simulink model "threelevel_12phase1"  (R2020b)
settings: Solver=FixedStepDiscrete  StartTime=0.0  StopTime=1  FixedStep=Ts_FEA  RelTol=1e-3
model workspace (MAT data in the model file):
  T_10kHz : Simulink.Parameter (value not decoded)
undefined symbols (not defined in the file): Cin, DiscIntNeverNeededParam, ESL, ESR, faif, Jm, kfeed_r, ki_n, kp_n, L, Ld, Line, Lq, ncmd_climb, ncmd_cruise, ncmd_run, ncmd_takeoff, p, Pcmd_climb, Pcmd_cruise, Pcmd_run, Pcmd_takeoff, Rs, Tcmd_run, Tcmd_start, Tcmd_time, time_climb, time_cruise, time_run, time_start, time_takeoff, Ts, Ts_Dead, Ts_FEA, Ts_speedloop, tswitch_climb, tswitch_takeoff, VDC, ws, zero_C1
libraries: powerlib x73, simulink x16, powerlib_meascontrol x16, slpidlib x13
(part 2 of 6)

== system threelevel_12phase1/CurrentLoop/Subsystem1/Subsystem ==
  ud : Inport
  uq : Inport  Port=2
  alpha : Inport  Port=3
  beta : Inport  Port=4
  dV : Inport  Port=5
  Atan2 : Trigonometry  Operator=atan2
  Constant : Constant
  Constant1 : Constant  Value=VDC
  Constant7 : Constant
  Divide : Product  Inputs=*/
  First_Order2 : Subsystem
  Gain : Gain  Gain=10
  PID Controller1 : slpidlib/PID Controller  Controller=PI  Form=Parallel  TimeDomain=Discrete-time  UseExternalTs=off  SampleTime=Ts  IntegratorMethod=Forward Euler  FilterMethod=Forward Euler  ControllerParametersSource=external  P=1/VDC  I=1/VDC  D=0  UseFilter=on  N=100  TunerSelectOption=Transfer Function Based (PID Tuner App)  InitialConditionSource=internal  InitialConditionForIntegrator=0  InitialConditionForFilter=0  DifferentiatorICPrevScaledInput=0  ExternalReset=none  TrackingMode=off  Kt=1  LimitOutput=on  SatLimitsSource=internal  UpperSaturationLimit=1  LowerSaturationLimit=-1  LinearizeAsGain=off  AntiWindupMode=none  Kb=1  POutMin=[]  POutMax=[]  IOutMin=[]  IOutMax=[]  DOutMin=[]  DOutMax=[]  NOutMin=[]  NOutMax=[]  SumOutMin=[]  SumOutMax=[]  SaturationOutMin=[]  SaturationOutMax=[]  PParamMin=[]  PParamMax=[]  IParamMin=[]  IParamMax=[]  DParamMin=[]  DParamMax=[]  NParamMin=[]  NParamMax=[]  KbParamMin=[]  KbParamMax=[]  KtParamMin=[]  KtParamMax=[]  KbOutMin=[]  KbOutMax=[]  KtOutMin=[]  KtOutMax=[]  IntegratorOutMin=[]  IntegratorOutMax=[]  FilterOutMin=[]  FilterOutMax=[]  SumI1OutMin=[]  SumI1OutMax=[]  SumI2OutMin=[]  SumI2OutMax=[]  SumI3OutMin=[]  SumI3OutMax=[]  SumI4OutMin=[]  SumI4OutMax=[]  SumDOutMin=[]  SumDOutMax=[]  DifferentiatorOutMin=[]  DifferentiatorOutMax=[]  FilterDiffOutCoefMin=[]  FilterDiffOutCoefMax=[]  ReciprocalOutMin=[]  ReciprocalOutMax=[]  SumDenOutMin=[]  SumDenOutMax=[]  SumNumOutMin=[]  SumNumOutMax=[]  DivideOutMin=[]  DivideOutMax=[]  UdiffTsProdOutMin=[]  UdiffTsProdOutMax=[]  NTsProdOutMin=[]  NTsProdOutMax=[]  UintegralTsProdOutMin=[]  UintegralTsProdOutMax=[]  UngainTsProdOutMin=[]  UngainTsProdOutMax=[]  IntegratorContinuousStateAttributes=''  IntegratorStateMustResolveToSignalObject=off  IntegratorRTWStateStorageClass=Auto  FilterContinuousStateAttributes=''  FilterStateMustResolveToSignalObject=off  FilterRTWStateStorageClass=Auto  ParallelPVariant=ExternalParameters  IdealPVariant=Disabled  IVariant=ExternalParameters  DVariant=Disabled  IntegratorVariant=Discrete  SatVariant=Enabled  AWVariant=Passthrough  PCopyVariant=Disabled  TRVariant=Disabled  FdbkBlocksVariant=Forward  IdealPFdbkVariant=Disabled  SatFdbkVariant=Disabled  DerivativeFilterVariant=Disabled  NVariant=Disabled  NCopyVariant=Disabled_SignalSpec  FilterICVariant=Disabled  IntegratorICVariant=InternalICs  ExternalResetVariant=Disabled  TRSumVariant=Passthrough  SumFdbkVariant=Disabled  SumVariant=Sum_PI  TsampFilterVariant=InternalTs  TsampNgainVariant=Passthrough  TsampIntegralVariant=Passthrough  ExternalSaturationOutDataTypeStr=Inherit: Same as second input
  Product1 : Product
  Saturation1 : Saturate  UpperLimit=1  LowerLimit=-1
  propose method1 : MATLAB Function  TreatAsAtomicUnit=on
  针对负载波动的P增量 : Subsystem  Commented=on
  r : Outport
  wires:
  Divide/1 -> Product1/1, Gain/1
  Constant1/1 -> Divide/2
  Constant7/1 -> Divide/1
  alpha/1 -> propose method1/2(alpha)
  uq/1 -> Atan2/2
  beta/1 -> propose method1/3(beta)
  propose method1/1(r) -> Saturation1/1
  Atan2/1 -> First_Order2/1(In1)
  ud/1 -> Atan2/1
  dV/1 -> PID Controller1/1
  Constant/1 -> Product1/2
  Gain/1 -> PID Controller1/3
  Product1/1 -> PID Controller1/2
  First_Order2/1(ADC_temp) -> propose method1/4(phi)
  Saturation1/1 -> r/1
  PID Controller1/1 -> propose method1/1(PI)

== system threelevel_12phase1/CurrentLoop/Subsystem1/Subsystem2 ==
  Compare : Inport
  AND13 : Logic  AllPortsSameDT=off  OutDataTypeStr=boolean
  AND14 : Logic  AllPortsSameDT=off  OutDataTypeStr=boolean
  Delay13 : Delay  DelayLength=Ts_Dead/Ts_FEA
  Demux : Demux  Outputs=6
  Demux1 : Demux  Outputs=6
  Mux : Mux  Inputs=12
  NOT6 : Logic  Operator=NOT  AllPortsSameDT=off  OutDataTypeStr=boolean
  NOT7 : Logic  Operator=NOT  AllPortsSameDT=off  OutDataTypeStr=boolean
  Output : Outport
  wires:
  Mux/1 -> Output/1
  Compare/1 -> Delay13/1, NOT6/1, AND13/1
  Delay13/1 -> NOT7/1, AND13/2
  NOT7/1 -> AND14/1
  NOT6/1 -> AND14/2
  AND13/1 -> Demux/1
  AND14/1 -> Demux1/1
  Demux/1 -> Mux/1
  Demux/2 -> Mux/2
  Demux/3 -> Mux/5
  Demux/4 -> Mux/6
  Demux/5 -> Mux/9
  Demux/6 -> Mux/10
  Demux1/1 -> Mux/3
  Demux1/2 -> Mux/4
  Demux1/3 -> Mux/7
  Demux1/4 -> Mux/8
  Demux1/5 -> Mux/11
  Demux1/6 -> Mux/12

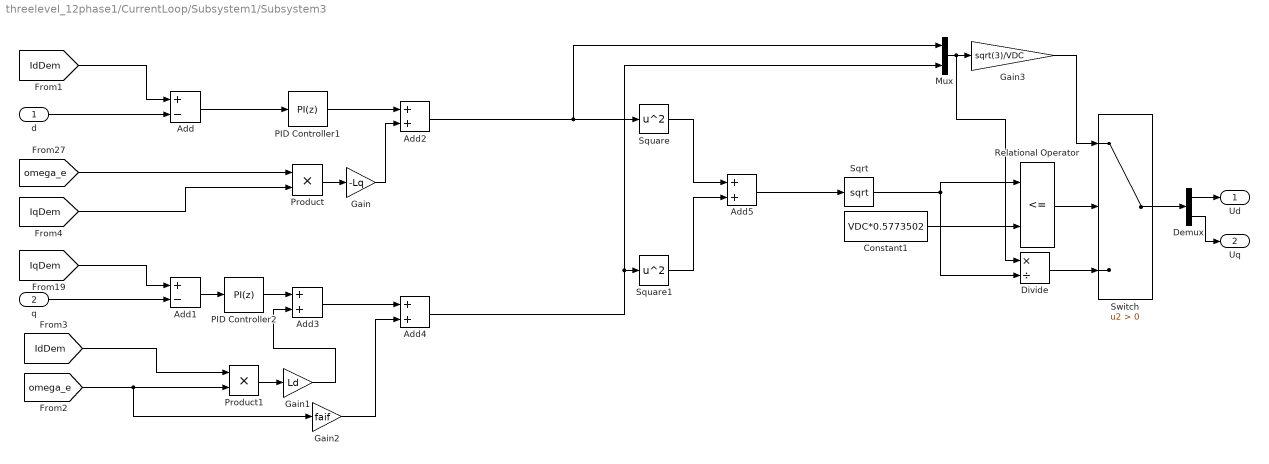
== system threelevel_12phase1/CurrentLoop/Subsystem1/Subsystem3 ==
  d : Inport
  q : Inport  Port=2
  Add : Sum  Inputs=+-
  Add1 : Sum  Inputs=+-
  Add{2..5} (4 alike) : Sum
  Constant1 : Constant  Value=VDC*0.5773502
  Demux : Demux  Outputs=2
  Divide : Product  Inputs=*/
  Gain : Gain  Gain=-Lq
  Gain1 : Gain  Gain=Ld
  Gain2 : Gain  Gain=faif
  Gain3 : Gain  Gain=sqrt(3)/VDC
  Mux : Mux  Inputs=2
  PID Controller1 : slpidlib/PID Controller  Controller=PI  Form=Parallel  TimeDomain=Discrete-time  UseExternalTs=off  SampleTime=Ts  IntegratorMethod=Forward Euler  FilterMethod=Forward Euler  ControllerParametersSource=internal  P=ws*2*pi*Ld  I=ws*2*pi*Rs  D=0  UseFilter=on  N=100  TunerSelectOption=Transfer Function Based (PID Tuner App)  InitialConditionSource=internal  InitialConditionForIntegrator=0  InitialConditionForFilter=0  DifferentiatorICPrevScaledInput=0  ExternalReset=none  TrackingMode=off  Kt=1  LimitOutput=off  SatLimitsSource=internal  UpperSaturationLimit=inf  LowerSaturationLimit=-inf  LinearizeAsGain=on  AntiWindupMode=none  Kb=1  POutMin=[]  POutMax=[]  IOutMin=[]  IOutMax=[]  DOutMin=[]  DOutMax=[]  NOutMin=[]  NOutMax=[]  SumOutMin=[]  SumOutMax=[]  SaturationOutMin=[]  SaturationOutMax=[]  PParamMin=[]  PParamMax=[]  IParamMin=[]  IParamMax=[]  DParamMin=[]  DParamMax=[]  NParamMin=[]  NParamMax=[]  KbParamMin=[]  KbParamMax=[]  KtParamMin=[]  KtParamMax=[]  KbOutMin=[]  KbOutMax=[]  KtOutMin=[]  KtOutMax=[]  IntegratorOutMin=[]  IntegratorOutMax=[]  FilterOutMin=[]  FilterOutMax=[]  SumI1OutMin=[]  SumI1OutMax=[]  SumI2OutMin=[]  SumI2OutMax=[]  SumI3OutMin=[]  SumI3OutMax=[]  SumI4OutMin=[]  SumI4OutMax=[]  SumDOutMin=[]  SumDOutMax=[]  DifferentiatorOutMin=[]  DifferentiatorOutMax=[]  FilterDiffOutCoefMin=[]  FilterDiffOutCoefMax=[]  ReciprocalOutMin=[]  ReciprocalOutMax=[]  SumDenOutMin=[]  SumDenOutMax=[]  SumNumOutMin=[]  SumNumOutMax=[]  DivideOutMin=[]  DivideOutMax=[]  UdiffTsProdOutMin=[]  UdiffTsProdOutMax=[]  NTsProdOutMin=[]  NTsProdOutMax=[]  UintegralTsProdOutMin=[]  UintegralTsProdOutMax=[]  UngainTsProdOutMin=[]  UngainTsProdOutMax=[]  IntegratorContinuousStateAttributes=''  IntegratorStateMustResolveToSignalObject=off  IntegratorRTWStateStorageClass=Auto  FilterContinuousStateAttributes=''  FilterStateMustResolveToSignalObject=off  FilterRTWStateStorageClass=Auto  ParallelPVariant=InternalParameters  IdealPVariant=Disabled  IVariant=InternalParameters  DVariant=Disabled  IntegratorVariant=Discrete  SatVariant=Disabled  AWVariant=Passthrough  PCopyVariant=Disabled  TRVariant=Disabled  FdbkBlocksVariant=Forward  IdealPFdbkVariant=Disabled  SatFdbkVariant=Disabled  DerivativeFilterVariant=Disabled  NVariant=Disabled  NCopyVariant=Disabled_SignalSpec  FilterICVariant=Disabled  IntegratorICVariant=InternalICs  ExternalResetVariant=Disabled  TRSumVariant=Passthrough  SumFdbkVariant=Disabled  SumVariant=Sum_PI  TsampFilterVariant=InternalTs  TsampNgainVariant=Passthrough  TsampIntegralVariant=Passthrough  ExternalSaturationOutDataTypeStr=Inherit: Same as second input
  PID Controller2 : slpidlib/PID Controller  Controller=PI  Form=Parallel  TimeDomain=Discrete-time  UseExternalTs=off  SampleTime=Ts  IntegratorMethod=Forward Euler  FilterMethod=Forward Euler  ControllerParametersSource=internal  P=ws*2*pi*Lq  I=ws*2*pi*Rs  D=0  UseFilter=on  N=100  TunerSelectOption=Transfer Function Based (PID Tuner App)  InitialConditionSource=internal  InitialConditionForIntegrator=0  InitialConditionForFilter=0  DifferentiatorICPrevScaledInput=0  ExternalReset=none  TrackingMode=off  Kt=1  LimitOutput=off  SatLimitsSource=internal  UpperSaturationLimit=inf  LowerSaturationLimit=-inf  LinearizeAsGain=on  AntiWindupMode=none  Kb=1  POutMin=[]  POutMax=[]  IOutMin=[]  IOutMax=[]  DOutMin=[]  DOutMax=[]  NOutMin=[]  NOutMax=[]  SumOutMin=[]  SumOutMax=[]  SaturationOutMin=[]  SaturationOutMax=[]  PParamMin=[]  PParamMax=[]  IParamMin=[]  IParamMax=[]  DParamMin=[]  DParamMax=[]  NParamMin=[]  NParamMax=[]  KbParamMin=[]  KbParamMax=[]  KtParamMin=[]  KtParamMax=[]  KbOutMin=[]  KbOutMax=[]  KtOutMin=[]  KtOutMax=[]  IntegratorOutMin=[]  IntegratorOutMax=[]  FilterOutMin=[]  FilterOutMax=[]  SumI1OutMin=[]  SumI1OutMax=[]  SumI2OutMin=[]  SumI2OutMax=[]  SumI3OutMin=[]  SumI3OutMax=[]  SumI4OutMin=[]  SumI4OutMax=[]  SumDOutMin=[]  SumDOutMax=[]  DifferentiatorOutMin=[]  DifferentiatorOutMax=[]  FilterDiffOutCoefMin=[]  FilterDiffOutCoefMax=[]  ReciprocalOutMin=[]  ReciprocalOutMax=[]  SumDenOutMin=[]  SumDenOutMax=[]  SumNumOutMin=[]  SumNumOutMax=[]  DivideOutMin=[]  DivideOutMax=[]  UdiffTsProdOutMin=[]  UdiffTsProdOutMax=[]  NTsProdOutMin=[]  NTsProdOutMax=[]  UintegralTsProdOutMin=[]  UintegralTsProdOutMax=[]  UngainTsProdOutMin=[]  UngainTsProdOutMax=[]  IntegratorContinuousStateAttributes=''  IntegratorStateMustResolveToSignalObject=off  IntegratorRTWStateStorageClass=Auto  FilterContinuousStateAttributes=''  FilterStateMustResolveToSignalObject=off  FilterRTWStateStorageClass=Auto  ParallelPVariant=InternalParameters  IdealPVariant=Disabled  IVariant=InternalParameters  DVariant=Disabled  IntegratorVariant=Discrete  SatVariant=Disabled  AWVariant=Passthrough  PCopyVariant=Disabled  TRVariant=Disabled  FdbkBlocksVariant=Forward  IdealPFdbkVariant=Disabled  SatFdbkVariant=Disabled  DerivativeFilterVariant=Disabled  NVariant=Disabled  NCopyVariant=Disabled_SignalSpec  FilterICVariant=Disabled  IntegratorICVariant=InternalICs  ExternalResetVariant=Disabled  TRSumVariant=Passthrough  SumFdbkVariant=Disabled  SumVariant=Sum_PI  TsampFilterVariant=InternalTs  TsampNgainVariant=Passthrough  TsampIntegralVariant=Passthrough  ExternalSaturationOutDataTypeStr=Inherit: Same as second input
  Product : Product
  Product1 : Product
  Relational Operator : RelationalOperator  Operator=<=  OutDataTypeStr=boolean  RndMeth=Simplest
  Sqrt : Sqrt  SaturateOnIntegerOverflow=on
  Square : Math  Operator=square  SaturateOnIntegerOverflow=on
  Square1 : Math  Operator=square  SaturateOnIntegerOverflow=on
  Switch : Switch  Criteria=u2 > Threshold
  Ud : Outport
  Uq : Outport  Port=2
  wires:
  d/1 -> Add/2
  q/1 -> Add1/2
  [IqDem] -> Add1/1
  Add/1 -> PID Controller1/1
  Add1/1 -> PID Controller2/1
  PID Controller1/1 -> Add2/1
  [omega_e] -> Product/1
  Product/1 -> Gain/1
  Gain/1 -> Add2/2
  PID Controller2/1 -> Add3/1
  Product1/1 -> Gain1/1
  Gain1/1 -> Add3/2
  Add3/1 -> Add4/1
  Gain2/1 -> Add4/2
  [omega_e] -> Gain2/1, Product1/2
  Add2/1 -> Square/1, Mux/1
  Add4/1 -> Mux/2, Square1/1
  Square/1 -> Add5/1
  Square1/1 -> Add5/2
  Sqrt/1 -> Relational Operator/1, Divide/2
  Constant1/1 -> Relational Operator/2
  Relational Operator/1 -> Switch/2
  Switch/1 -> Demux/1
  Demux/1 -> Ud/1
  Demux/2 -> Uq/1
  Mux/1 -> Divide/1, Gain3/1
  Gain3/1 -> Switch/1
  Divide/1 -> Switch/3
  [IdDem] -> Add/1
  [IdDem] -> Product1/1
  [IqDem] -> Product/2
  Add5/1 -> Sqrt/1

== system threelevel_12phase1/CurrentLoop/Subsystem2/Subsystem ==
  ud : Inport
  uq : Inport  Port=2
  alpha : Inport  Port=3
  beta : Inport  Port=4
  dV : Inport  Port=5
  Atan2 : Trigonometry  Operator=atan2
  Constant : Constant
  Constant1 : Constant  Value=VDC
  Constant7 : Constant
  Divide : Product  Inputs=*/
  First_Order2 : Subsystem
  Gain : Gain  Gain=10
  PID Controller1 : slpidlib/PID Controller  Controller=PI  Form=Parallel  TimeDomain=Discrete-time  UseExternalTs=off  SampleTime=Ts  IntegratorMethod=Forward Euler  FilterMethod=Forward Euler  ControllerParametersSource=external  P=1/VDC  I=1/VDC  D=0  UseFilter=on  N=100  TunerSelectOption=Transfer Function Based (PID Tuner App)  InitialConditionSource=internal  InitialConditionForIntegrator=0  InitialConditionForFilter=0  DifferentiatorICPrevScaledInput=0  ExternalReset=none  TrackingMode=off  Kt=1  LimitOutput=on  SatLimitsSource=internal  UpperSaturationLimit=1  LowerSaturationLimit=-1  LinearizeAsGain=off  AntiWindupMode=none  Kb=1  POutMin=[]  POutMax=[]  IOutMin=[]  IOutMax=[]  DOutMin=[]  DOutMax=[]  NOutMin=[]  NOutMax=[]  SumOutMin=[]  SumOutMax=[]  SaturationOutMin=[]  SaturationOutMax=[]  PParamMin=[]  PParamMax=[]  IParamMin=[]  IParamMax=[]  DParamMin=[]  DParamMax=[]  NParamMin=[]  NParamMax=[]  KbParamMin=[]  KbParamMax=[]  KtParamMin=[]  KtParamMax=[]  KbOutMin=[]  KbOutMax=[]  KtOutMin=[]  KtOutMax=[]  IntegratorOutMin=[]  IntegratorOutMax=[]  FilterOutMin=[]  FilterOutMax=[]  SumI1OutMin=[]  SumI1OutMax=[]  SumI2OutMin=[]  SumI2OutMax=[]  SumI3OutMin=[]  SumI3OutMax=[]  SumI4OutMin=[]  SumI4OutMax=[]  SumDOutMin=[]  SumDOutMax=[]  DifferentiatorOutMin=[]  DifferentiatorOutMax=[]  FilterDiffOutCoefMin=[]  FilterDiffOutCoefMax=[]  ReciprocalOutMin=[]  ReciprocalOutMax=[]  SumDenOutMin=[]  SumDenOutMax=[]  SumNumOutMin=[]  SumNumOutMax=[]  DivideOutMin=[]  DivideOutMax=[]  UdiffTsProdOutMin=[]  UdiffTsProdOutMax=[]  NTsProdOutMin=[]  NTsProdOutMax=[]  UintegralTsProdOutMin=[]  UintegralTsProdOutMax=[]  UngainTsProdOutMin=[]  UngainTsProdOutMax=[]  IntegratorContinuousStateAttributes=''  IntegratorStateMustResolveToSignalObject=off  IntegratorRTWStateStorageClass=Auto  FilterContinuousStateAttributes=''  FilterStateMustResolveToSignalObject=off  FilterRTWStateStorageClass=Auto  ParallelPVariant=ExternalParameters  IdealPVariant=Disabled  IVariant=ExternalParameters  DVariant=Disabled  IntegratorVariant=Discrete  SatVariant=Enabled  AWVariant=Passthrough  PCopyVariant=Disabled  TRVariant=Disabled  FdbkBlocksVariant=Forward  IdealPFdbkVariant=Disabled  SatFdbkVariant=Disabled  DerivativeFilterVariant=Disabled  NVariant=Disabled  NCopyVariant=Disabled_SignalSpec  FilterICVariant=Disabled  IntegratorICVariant=InternalICs  ExternalResetVariant=Disabled  TRSumVariant=Passthrough  SumFdbkVariant=Disabled  SumVariant=Sum_PI  TsampFilterVariant=InternalTs  TsampNgainVariant=Passthrough  TsampIntegralVariant=Passthrough  ExternalSaturationOutDataTypeStr=Inherit: Same as second input
  Product1 : Product
  Saturation1 : Saturate  UpperLimit=1  LowerLimit=-1
  propose method1 : MATLAB Function  TreatAsAtomicUnit=on
  针对负载波动的P增量 : Subsystem  Commented=on
  r : Outport
  wires:
  Divide/1 -> Product1/1, Gain/1
  Constant1/1 -> Divide/2
  Constant7/1 -> Divide/1
  alpha/1 -> propose method1/2(alpha)
  uq/1 -> Atan2/2
  beta/1 -> propose method1/3(beta)
  propose method1/1(r) -> Saturation1/1
  Atan2/1 -> First_Order2/1(In1)
  ud/1 -> Atan2/1
  dV/1 -> PID Controller1/1
  Constant/1 -> Product1/2
  Gain/1 -> PID Controller1/3
  Product1/1 -> PID Controller1/2
  First_Order2/1(ADC_temp) -> propose method1/4(phi)
  Saturation1/1 -> r/1
  PID Controller1/1 -> propose method1/1(PI)

== system threelevel_12phase1/CurrentLoop/Subsystem2/Subsystem2 ==
  Compare : Inport
  AND13 : Logic  AllPortsSameDT=off  OutDataTypeStr=boolean
  AND14 : Logic  AllPortsSameDT=off  OutDataTypeStr=boolean
  Delay13 : Delay  DelayLength=Ts_Dead/Ts_FEA
  Demux : Demux  Outputs=6
  Demux1 : Demux  Outputs=6
  Mux : Mux  Inputs=12
  NOT6 : Logic  Operator=NOT  AllPortsSameDT=off  OutDataTypeStr=boolean
  NOT7 : Logic  Operator=NOT  AllPortsSameDT=off  OutDataTypeStr=boolean
  Output : Outport
  wires:
  Mux/1 -> Output/1
  Compare/1 -> Delay13/1, NOT6/1, AND13/1
  Delay13/1 -> NOT7/1, AND13/2
  NOT7/1 -> AND14/1
  NOT6/1 -> AND14/2
  AND13/1 -> Demux/1
  AND14/1 -> Demux1/1
  Demux/1 -> Mux/1
  Demux/2 -> Mux/2
  Demux/3 -> Mux/5
  Demux/4 -> Mux/6
  Demux/5 -> Mux/9
  Demux/6 -> Mux/10
  Demux1/1 -> Mux/3
  Demux1/2 -> Mux/4
  Demux1/3 -> Mux/7
  Demux1/4 -> Mux/8
  Demux1/5 -> Mux/11
  Demux1/6 -> Mux/12

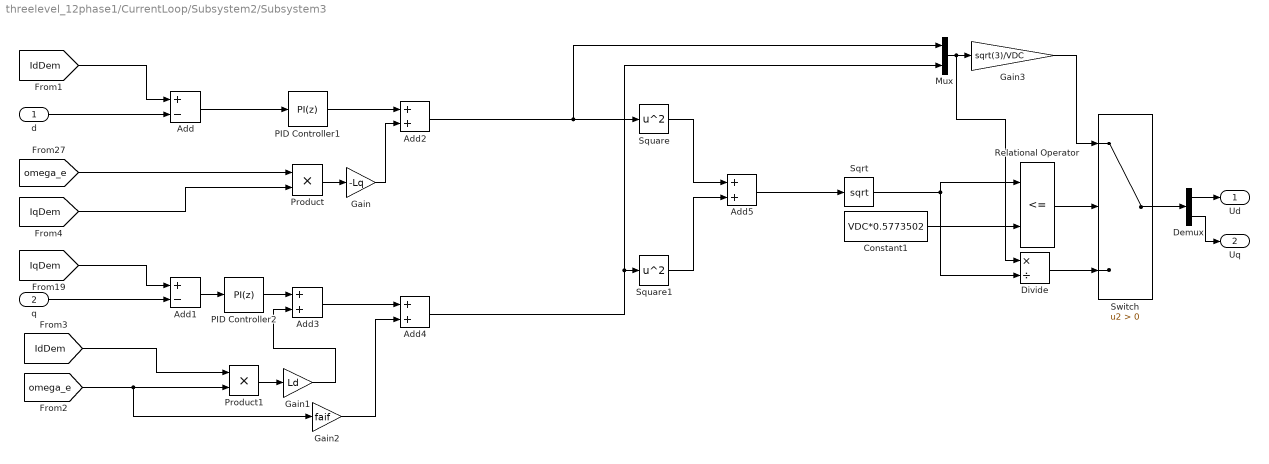
== system threelevel_12phase1/CurrentLoop/Subsystem2/Subsystem3 ==
  d : Inport
  q : Inport  Port=2
  Add : Sum  Inputs=+-
  Add1 : Sum  Inputs=+-
  Add{2..5} (4 alike) : Sum
  Constant1 : Constant  Value=VDC*0.5773502
  Demux : Demux  Outputs=2
  Divide : Product  Inputs=*/
  Gain : Gain  Gain=-Lq
  Gain1 : Gain  Gain=Ld
  Gain2 : Gain  Gain=faif
  Gain3 : Gain  Gain=sqrt(3)/VDC
  Mux : Mux  Inputs=2
  PID Controller1 : slpidlib/PID Controller  Controller=PI  Form=Parallel  TimeDomain=Discrete-time  UseExternalTs=off  SampleTime=Ts  IntegratorMethod=Forward Euler  FilterMethod=Forward Euler  ControllerParametersSource=internal  P=ws*2*pi*Ld  I=ws*2*pi*Rs  D=0  UseFilter=on  N=100  TunerSelectOption=Transfer Function Based (PID Tuner App)  InitialConditionSource=internal  InitialConditionForIntegrator=0  InitialConditionForFilter=0  DifferentiatorICPrevScaledInput=0  ExternalReset=none  TrackingMode=off  Kt=1  LimitOutput=off  SatLimitsSource=internal  UpperSaturationLimit=inf  LowerSaturationLimit=-inf  LinearizeAsGain=on  AntiWindupMode=none  Kb=1  POutMin=[]  POutMax=[]  IOutMin=[]  IOutMax=[]  DOutMin=[]  DOutMax=[]  NOutMin=[]  NOutMax=[]  SumOutMin=[]  SumOutMax=[]  SaturationOutMin=[]  SaturationOutMax=[]  PParamMin=[]  PParamMax=[]  IParamMin=[]  IParamMax=[]  DParamMin=[]  DParamMax=[]  NParamMin=[]  NParamMax=[]  KbParamMin=[]  KbParamMax=[]  KtParamMin=[]  KtParamMax=[]  KbOutMin=[]  KbOutMax=[]  KtOutMin=[]  KtOutMax=[]  IntegratorOutMin=[]  IntegratorOutMax=[]  FilterOutMin=[]  FilterOutMax=[]  SumI1OutMin=[]  SumI1OutMax=[]  SumI2OutMin=[]  SumI2OutMax=[]  SumI3OutMin=[]  SumI3OutMax=[]  SumI4OutMin=[]  SumI4OutMax=[]  SumDOutMin=[]  SumDOutMax=[]  DifferentiatorOutMin=[]  DifferentiatorOutMax=[]  FilterDiffOutCoefMin=[]  FilterDiffOutCoefMax=[]  ReciprocalOutMin=[]  ReciprocalOutMax=[]  SumDenOutMin=[]  SumDenOutMax=[]  SumNumOutMin=[]  SumNumOutMax=[]  DivideOutMin=[]  DivideOutMax=[]  UdiffTsProdOutMin=[]  UdiffTsProdOutMax=[]  NTsProdOutMin=[]  NTsProdOutMax=[]  UintegralTsProdOutMin=[]  UintegralTsProdOutMax=[]  UngainTsProdOutMin=[]  UngainTsProdOutMax=[]  IntegratorContinuousStateAttributes=''  IntegratorStateMustResolveToSignalObject=off  IntegratorRTWStateStorageClass=Auto  FilterContinuousStateAttributes=''  FilterStateMustResolveToSignalObject=off  FilterRTWStateStorageClass=Auto  ParallelPVariant=InternalParameters  IdealPVariant=Disabled  IVariant=InternalParameters  DVariant=Disabled  IntegratorVariant=Discrete  SatVariant=Disabled  AWVariant=Passthrough  PCopyVariant=Disabled  TRVariant=Disabled  FdbkBlocksVariant=Forward  IdealPFdbkVariant=Disabled  SatFdbkVariant=Disabled  DerivativeFilterVariant=Disabled  NVariant=Disabled  NCopyVariant=Disabled_SignalSpec  FilterICVariant=Disabled  IntegratorICVariant=InternalICs  ExternalResetVariant=Disabled  TRSumVariant=Passthrough  SumFdbkVariant=Disabled  SumVariant=Sum_PI  TsampFilterVariant=InternalTs  TsampNgainVariant=Passthrough  TsampIntegralVariant=Passthrough  ExternalSaturationOutDataTypeStr=Inherit: Same as second input
  PID Controller2 : slpidlib/PID Controller  Controller=PI  Form=Parallel  TimeDomain=Discrete-time  UseExternalTs=off  SampleTime=Ts  IntegratorMethod=Forward Euler  FilterMethod=Forward Euler  ControllerParametersSource=internal  P=ws*2*pi*Lq  I=ws*2*pi*Rs  D=0  UseFilter=on  N=100  TunerSelectOption=Transfer Function Based (PID Tuner App)  InitialConditionSource=internal  InitialConditionForIntegrator=0  InitialConditionForFilter=0  DifferentiatorICPrevScaledInput=0  ExternalReset=none  TrackingMode=off  Kt=1  LimitOutput=off  SatLimitsSource=internal  UpperSaturationLimit=inf  LowerSaturationLimit=-inf  LinearizeAsGain=on  AntiWindupMode=none  Kb=1  POutMin=[]  POutMax=[]  IOutMin=[]  IOutMax=[]  DOutMin=[]  DOutMax=[]  NOutMin=[]  NOutMax=[]  SumOutMin=[]  SumOutMax=[]  SaturationOutMin=[]  SaturationOutMax=[]  PParamMin=[]  PParamMax=[]  IParamMin=[]  IParamMax=[]  DParamMin=[]  DParamMax=[]  NParamMin=[]  NParamMax=[]  KbParamMin=[]  KbParamMax=[]  KtParamMin=[]  KtParamMax=[]  KbOutMin=[]  KbOutMax=[]  KtOutMin=[]  KtOutMax=[]  IntegratorOutMin=[]  IntegratorOutMax=[]  FilterOutMin=[]  FilterOutMax=[]  SumI1OutMin=[]  SumI1OutMax=[]  SumI2OutMin=[]  SumI2OutMax=[]  SumI3OutMin=[]  SumI3OutMax=[]  SumI4OutMin=[]  SumI4OutMax=[]  SumDOutMin=[]  SumDOutMax=[]  DifferentiatorOutMin=[]  DifferentiatorOutMax=[]  FilterDiffOutCoefMin=[]  FilterDiffOutCoefMax=[]  ReciprocalOutMin=[]  ReciprocalOutMax=[]  SumDenOutMin=[]  SumDenOutMax=[]  SumNumOutMin=[]  SumNumOutMax=[]  DivideOutMin=[]  DivideOutMax=[]  UdiffTsProdOutMin=[]  UdiffTsProdOutMax=[]  NTsProdOutMin=[]  NTsProdOutMax=[]  UintegralTsProdOutMin=[]  UintegralTsProdOutMax=[]  UngainTsProdOutMin=[]  UngainTsProdOutMax=[]  IntegratorContinuousStateAttributes=''  IntegratorStateMustResolveToSignalObject=off  IntegratorRTWStateStorageClass=Auto  FilterContinuousStateAttributes=''  FilterStateMustResolveToSignalObject=off  FilterRTWStateStorageClass=Auto  ParallelPVariant=InternalParameters  IdealPVariant=Disabled  IVariant=InternalParameters  DVariant=Disabled  IntegratorVariant=Discrete  SatVariant=Disabled  AWVariant=Passthrough  PCopyVariant=Disabled  TRVariant=Disabled  FdbkBlocksVariant=Forward  IdealPFdbkVariant=Disabled  SatFdbkVariant=Disabled  DerivativeFilterVariant=Disabled  NVariant=Disabled  NCopyVariant=Disabled_SignalSpec  FilterICVariant=Disabled  IntegratorICVariant=InternalICs  ExternalResetVariant=Disabled  TRSumVariant=Passthrough  SumFdbkVariant=Disabled  SumVariant=Sum_PI  TsampFilterVariant=InternalTs  TsampNgainVariant=Passthrough  TsampIntegralVariant=Passthrough  ExternalSaturationOutDataTypeStr=Inherit: Same as second input
  Product : Product
  Product1 : Product
  Relational Operator : RelationalOperator  Operator=<=  OutDataTypeStr=boolean  RndMeth=Simplest
  Sqrt : Sqrt  SaturateOnIntegerOverflow=on
  Square : Math  Operator=square  SaturateOnIntegerOverflow=on
  Square1 : Math  Operator=square  SaturateOnIntegerOverflow=on
  Switch : Switch  Criteria=u2 > Threshold
  Ud : Outport
  Uq : Outport  Port=2
  wires:
  d/1 -> Add/2
  q/1 -> Add1/2
  [IqDem] -> Add1/1
  Add/1 -> PID Controller1/1
  Add1/1 -> PID Controller2/1
  PID Controller1/1 -> Add2/1
  [omega_e] -> Product/1
  Product/1 -> Gain/1
  Gain/1 -> Add2/2
  PID Controller2/1 -> Add3/1
  Product1/1 -> Gain1/1
  Gain1/1 -> Add3/2
  Add3/1 -> Add4/1
  Gain2/1 -> Add4/2
  [omega_e] -> Gain2/1, Product1/2
  Add2/1 -> Square/1, Mux/1
  Add4/1 -> Mux/2, Square1/1
  Square/1 -> Add5/1
  Square1/1 -> Add5/2
  Sqrt/1 -> Relational Operator/1, Divide/2
  Constant1/1 -> Relational Operator/2
  Relational Operator/1 -> Switch/2
  Switch/1 -> Demux/1
  Demux/1 -> Ud/1
  Demux/2 -> Uq/1
  Mux/1 -> Divide/1, Gain3/1
  Gain3/1 -> Switch/1
  Divide/1 -> Switch/3
  [IdDem] -> Add/1
  [IdDem] -> Product1/1
  [IqDem] -> Product/2
  Add5/1 -> Sqrt/1

== system threelevel_12phase1/CurrentLoop/Subsystem3/Subsystem ==
  ud : Inport
  uq : Inport  Port=2
  alpha : Inport  Port=3
  beta : Inport  Port=4
  dV : Inport  Port=5
  Atan2 : Trigonometry  Operator=atan2
  Constant : Constant
  Constant1 : Constant  Value=VDC
  Constant7 : Constant
  Divide : Product  Inputs=*/
  First_Order2 : Subsystem
  Gain : Gain  Gain=10
  PID Controller1 : slpidlib/PID Controller  Controller=PI  Form=Parallel  TimeDomain=Discrete-time  UseExternalTs=off  SampleTime=Ts  IntegratorMethod=Forward Euler  FilterMethod=Forward Euler  ControllerParametersSource=external  P=1/VDC  I=1/VDC  D=0  UseFilter=on  N=100  TunerSelectOption=Transfer Function Based (PID Tuner App)  InitialConditionSource=internal  InitialConditionForIntegrator=0  InitialConditionForFilter=0  DifferentiatorICPrevScaledInput=0  ExternalReset=none  TrackingMode=off  Kt=1  LimitOutput=on  SatLimitsSource=internal  UpperSaturationLimit=1  LowerSaturationLimit=-1  LinearizeAsGain=off  AntiWindupMode=none  Kb=1  POutMin=[]  POutMax=[]  IOutMin=[]  IOutMax=[]  DOutMin=[]  DOutMax=[]  NOutMin=[]  NOutMax=[]  SumOutMin=[]  SumOutMax=[]  SaturationOutMin=[]  SaturationOutMax=[]  PParamMin=[]  PParamMax=[]  IParamMin=[]  IParamMax=[]  DParamMin=[]  DParamMax=[]  NParamMin=[]  NParamMax=[]  KbParamMin=[]  KbParamMax=[]  KtParamMin=[]  KtParamMax=[]  KbOutMin=[]  KbOutMax=[]  KtOutMin=[]  KtOutMax=[]  IntegratorOutMin=[]  IntegratorOutMax=[]  FilterOutMin=[]  FilterOutMax=[]  SumI1OutMin=[]  SumI1OutMax=[]  SumI2OutMin=[]  SumI2OutMax=[]  SumI3OutMin=[]  SumI3OutMax=[]  SumI4OutMin=[]  SumI4OutMax=[]  SumDOutMin=[]  SumDOutMax=[]  DifferentiatorOutMin=[]  DifferentiatorOutMax=[]  FilterDiffOutCoefMin=[]  FilterDiffOutCoefMax=[]  ReciprocalOutMin=[]  ReciprocalOutMax=[]  SumDenOutMin=[]  SumDenOutMax=[]  SumNumOutMin=[]  SumNumOutMax=[]  DivideOutMin=[]  DivideOutMax=[]  UdiffTsProdOutMin=[]  UdiffTsProdOutMax=[]  NTsProdOutMin=[]  NTsProdOutMax=[]  UintegralTsProdOutMin=[]  UintegralTsProdOutMax=[]  UngainTsProdOutMin=[]  UngainTsProdOutMax=[]  IntegratorContinuousStateAttributes=''  IntegratorStateMustResolveToSignalObject=off  IntegratorRTWStateStorageClass=Auto  FilterContinuousStateAttributes=''  FilterStateMustResolveToSignalObject=off  FilterRTWStateStorageClass=Auto  ParallelPVariant=ExternalParameters  IdealPVariant=Disabled  IVariant=ExternalParameters  DVariant=Disabled  IntegratorVariant=Discrete  SatVariant=Enabled  AWVariant=Passthrough  PCopyVariant=Disabled  TRVariant=Disabled  FdbkBlocksVariant=Forward  IdealPFdbkVariant=Disabled  SatFdbkVariant=Disabled  DerivativeFilterVariant=Disabled  NVariant=Disabled  NCopyVariant=Disabled_SignalSpec  FilterICVariant=Disabled  IntegratorICVariant=InternalICs  ExternalResetVariant=Disabled  TRSumVariant=Passthrough  SumFdbkVariant=Disabled  SumVariant=Sum_PI  TsampFilterVariant=InternalTs  TsampNgainVariant=Passthrough  TsampIntegralVariant=Passthrough  ExternalSaturationOutDataTypeStr=Inherit: Same as second input
  Product1 : Product
  Saturation1 : Saturate  UpperLimit=1  LowerLimit=-1
  propose method1 : MATLAB Function  TreatAsAtomicUnit=on
  针对负载波动的P增量 : Subsystem  Commented=on
  r : Outport
  wires:
  Divide/1 -> Product1/1, Gain/1
  Constant1/1 -> Divide/2
  Constant7/1 -> Divide/1
  alpha/1 -> propose method1/2(alpha)
  uq/1 -> Atan2/2
  beta/1 -> propose method1/3(beta)
  propose method1/1(r) -> Saturation1/1
  Atan2/1 -> First_Order2/1(In1)
  ud/1 -> Atan2/1
  dV/1 -> PID Controller1/1
  Constant/1 -> Product1/2
  Gain/1 -> PID Controller1/3
  Product1/1 -> PID Controller1/2
  First_Order2/1(ADC_temp) -> propose method1/4(phi)
  Saturation1/1 -> r/1
  PID Controller1/1 -> propose method1/1(PI)

== system threelevel_12phase1/CurrentLoop/Subsystem3/Subsystem2 ==
  Compare : Inport
  AND13 : Logic  AllPortsSameDT=off  OutDataTypeStr=boolean
  AND14 : Logic  AllPortsSameDT=off  OutDataTypeStr=boolean
  Delay13 : Delay  DelayLength=Ts_Dead/Ts_FEA
  Demux : Demux  Outputs=6
  Demux1 : Demux  Outputs=6
  Mux : Mux  Inputs=12
  NOT6 : Logic  Operator=NOT  AllPortsSameDT=off  OutDataTypeStr=boolean
  NOT7 : Logic  Operator=NOT  AllPortsSameDT=off  OutDataTypeStr=boolean
  Output : Outport
  wires:
  Mux/1 -> Output/1
  Compare/1 -> Delay13/1, NOT6/1, AND13/1
  Delay13/1 -> NOT7/1, AND13/2
  NOT7/1 -> AND14/1
  NOT6/1 -> AND14/2
  AND13/1 -> Demux/1
  AND14/1 -> Demux1/1
  Demux/1 -> Mux/1
  Demux/2 -> Mux/2
  Demux/3 -> Mux/5
  Demux/4 -> Mux/6
  Demux/5 -> Mux/9
  Demux/6 -> Mux/10
  Demux1/1 -> Mux/3
  Demux1/2 -> Mux/4
  Demux1/3 -> Mux/7
  Demux1/4 -> Mux/8
  Demux1/5 -> Mux/11
  Demux1/6 -> Mux/12

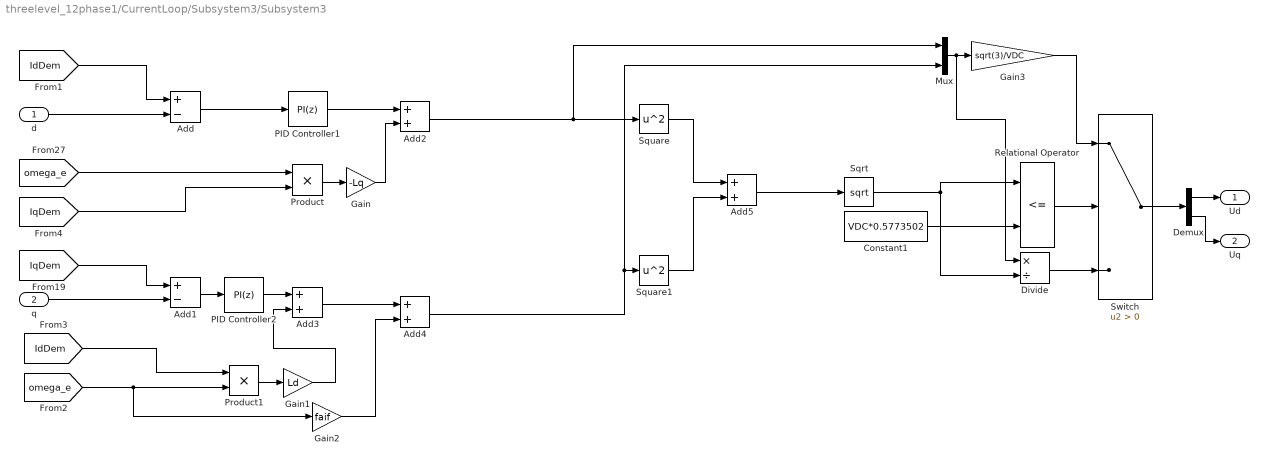
== system threelevel_12phase1/CurrentLoop/Subsystem3/Subsystem3 ==
  d : Inport
  q : Inport  Port=2
  Add : Sum  Inputs=+-
  Add1 : Sum  Inputs=+-
  Add{2..5} (4 alike) : Sum
  Constant1 : Constant  Value=VDC*0.5773502
  Demux : Demux  Outputs=2
  Divide : Product  Inputs=*/
  Gain : Gain  Gain=-Lq
  Gain1 : Gain  Gain=Ld
  Gain2 : Gain  Gain=faif
  Gain3 : Gain  Gain=sqrt(3)/VDC
  Mux : Mux  Inputs=2
  PID Controller1 : slpidlib/PID Controller  Controller=PI  Form=Parallel  TimeDomain=Discrete-time  UseExternalTs=off  SampleTime=Ts  IntegratorMethod=Forward Euler  FilterMethod=Forward Euler  ControllerParametersSource=internal  P=ws*2*pi*Ld  I=ws*2*pi*Rs  D=0  UseFilter=on  N=100  TunerSelectOption=Transfer Function Based (PID Tuner App)  InitialConditionSource=internal  InitialConditionForIntegrator=0  InitialConditionForFilter=0  DifferentiatorICPrevScaledInput=0  ExternalReset=none  TrackingMode=off  Kt=1  LimitOutput=off  SatLimitsSource=internal  UpperSaturationLimit=inf  LowerSaturationLimit=-inf  LinearizeAsGain=on  AntiWindupMode=none  Kb=1  POutMin=[]  POutMax=[]  IOutMin=[]  IOutMax=[]  DOutMin=[]  DOutMax=[]  NOutMin=[]  NOutMax=[]  SumOutMin=[]  SumOutMax=[]  SaturationOutMin=[]  SaturationOutMax=[]  PParamMin=[]  PParamMax=[]  IParamMin=[]  IParamMax=[]  DParamMin=[]  DParamMax=[]  NParamMin=[]  NParamMax=[]  KbParamMin=[]  KbParamMax=[]  KtParamMin=[]  KtParamMax=[]  KbOutMin=[]  KbOutMax=[]  KtOutMin=[]  KtOutMax=[]  IntegratorOutMin=[]  IntegratorOutMax=[]  FilterOutMin=[]  FilterOutMax=[]  SumI1OutMin=[]  SumI1OutMax=[]  SumI2OutMin=[]  SumI2OutMax=[]  SumI3OutMin=[]  SumI3OutMax=[]  SumI4OutMin=[]  SumI4OutMax=[]  SumDOutMin=[]  SumDOutMax=[]  DifferentiatorOutMin=[]  DifferentiatorOutMax=[]  FilterDiffOutCoefMin=[]  FilterDiffOutCoefMax=[]  ReciprocalOutMin=[]  ReciprocalOutMax=[]  SumDenOutMin=[]  SumDenOutMax=[]  SumNumOutMin=[]  SumNumOutMax=[]  DivideOutMin=[]  DivideOutMax=[]  UdiffTsProdOutMin=[]  UdiffTsProdOutMax=[]  NTsProdOutMin=[]  NTsProdOutMax=[]  UintegralTsProdOutMin=[]  UintegralTsProdOutMax=[]  UngainTsProdOutMin=[]  UngainTsProdOutMax=[]  IntegratorContinuousStateAttributes=''  IntegratorStateMustResolveToSignalObject=off  IntegratorRTWStateStorageClass=Auto  FilterContinuousStateAttributes=''  FilterStateMustResolveToSignalObject=off  FilterRTWStateStorageClass=Auto  ParallelPVariant=InternalParameters  IdealPVariant=Disabled  IVariant=InternalParameters  DVariant=Disabled  IntegratorVariant=Discrete  SatVariant=Disabled  AWVariant=Passthrough  PCopyVariant=Disabled  TRVariant=Disabled  FdbkBlocksVariant=Forward  IdealPFdbkVariant=Disabled  SatFdbkVariant=Disabled  DerivativeFilterVariant=Disabled  NVariant=Disabled  NCopyVariant=Disabled_SignalSpec  FilterICVariant=Disabled  IntegratorICVariant=InternalICs  ExternalResetVariant=Disabled  TRSumVariant=Passthrough  SumFdbkVariant=Disabled  SumVariant=Sum_PI  TsampFilterVariant=InternalTs  TsampNgainVariant=Passthrough  TsampIntegralVariant=Passthrough  ExternalSaturationOutDataTypeStr=Inherit: Same as second input
  PID Controller2 : slpidlib/PID Controller  Controller=PI  Form=Parallel  TimeDomain=Discrete-time  UseExternalTs=off  SampleTime=Ts  IntegratorMethod=Forward Euler  FilterMethod=Forward Euler  ControllerParametersSource=internal  P=ws*2*pi*Lq  I=ws*2*pi*Rs  D=0  UseFilter=on  N=100  TunerSelectOption=Transfer Function Based (PID Tuner App)  InitialConditionSource=internal  InitialConditionForIntegrator=0  InitialConditionForFilter=0  DifferentiatorICPrevScaledInput=0  ExternalReset=none  TrackingMode=off  Kt=1  LimitOutput=off  SatLimitsSource=internal  UpperSaturationLimit=inf  LowerSaturationLimit=-inf  LinearizeAsGain=on  AntiWindupMode=none  Kb=1  POutMin=[]  POutMax=[]  IOutMin=[]  IOutMax=[]  DOutMin=[]  DOutMax=[]  NOutMin=[]  NOutMax=[]  SumOutMin=[]  SumOutMax=[]  SaturationOutMin=[]  SaturationOutMax=[]  PParamMin=[]  PParamMax=[]  IParamMin=[]  IParamMax=[]  DParamMin=[]  DParamMax=[]  NParamMin=[]  NParamMax=[]  KbParamMin=[]  KbParamMax=[]  KtParamMin=[]  KtParamMax=[]  KbOutMin=[]  KbOutMax=[]  KtOutMin=[]  KtOutMax=[]  IntegratorOutMin=[]  IntegratorOutMax=[]  FilterOutMin=[]  FilterOutMax=[]  SumI1OutMin=[]  SumI1OutMax=[]  SumI2OutMin=[]  SumI2OutMax=[]  SumI3OutMin=[]  SumI3OutMax=[]  SumI4OutMin=[]  SumI4OutMax=[]  SumDOutMin=[]  SumDOutMax=[]  DifferentiatorOutMin=[]  DifferentiatorOutMax=[]  FilterDiffOutCoefMin=[]  FilterDiffOutCoefMax=[]  ReciprocalOutMin=[]  ReciprocalOutMax=[]  SumDenOutMin=[]  SumDenOutMax=[]  SumNumOutMin=[]  SumNumOutMax=[]  DivideOutMin=[]  DivideOutMax=[]  UdiffTsProdOutMin=[]  UdiffTsProdOutMax=[]  NTsProdOutMin=[]  NTsProdOutMax=[]  UintegralTsProdOutMin=[]  UintegralTsProdOutMax=[]  UngainTsProdOutMin=[]  UngainTsProdOutMax=[]  IntegratorContinuousStateAttributes=''  IntegratorStateMustResolveToSignalObject=off  IntegratorRTWStateStorageClass=Auto  FilterContinuousStateAttributes=''  FilterStateMustResolveToSignalObject=off  FilterRTWStateStorageClass=Auto  ParallelPVariant=InternalParameters  IdealPVariant=Disabled  IVariant=InternalParameters  DVariant=Disabled  IntegratorVariant=Discrete  SatVariant=Disabled  AWVariant=Passthrough  PCopyVariant=Disabled  TRVariant=Disabled  FdbkBlocksVariant=Forward  IdealPFdbkVariant=Disabled  SatFdbkVariant=Disabled  DerivativeFilterVariant=Disabled  NVariant=Disabled  NCopyVariant=Disabled_SignalSpec  FilterICVariant=Disabled  IntegratorICVariant=InternalICs  ExternalResetVariant=Disabled  TRSumVariant=Passthrough  SumFdbkVariant=Disabled  SumVariant=Sum_PI  TsampFilterVariant=InternalTs  TsampNgainVariant=Passthrough  TsampIntegralVariant=Passthrough  ExternalSaturationOutDataTypeStr=Inherit: Same as second input
  Product : Product
  Product1 : Product
  Relational Operator : RelationalOperator  Operator=<=  OutDataTypeStr=boolean  RndMeth=Simplest
  Sqrt : Sqrt  SaturateOnIntegerOverflow=on
  Square : Math  Operator=square  SaturateOnIntegerOverflow=on
  Square1 : Math  Operator=square  SaturateOnIntegerOverflow=on
  Switch : Switch  Criteria=u2 > Threshold
  Ud : Outport
  Uq : Outport  Port=2
  wires:
  d/1 -> Add/2
  q/1 -> Add1/2
  [IqDem] -> Add1/1
  Add/1 -> PID Controller1/1
  Add1/1 -> PID Controller2/1
  PID Controller1/1 -> Add2/1
  [omega_e] -> Product/1
  Product/1 -> Gain/1
  Gain/1 -> Add2/2
  PID Controller2/1 -> Add3/1
  Product1/1 -> Gain1/1
  Gain1/1 -> Add3/2
  Add3/1 -> Add4/1
  Gain2/1 -> Add4/2
  [omega_e] -> Gain2/1, Product1/2
  Add2/1 -> Square/1, Mux/1
  Add4/1 -> Mux/2, Square1/1
  Square/1 -> Add5/1
  Square1/1 -> Add5/2
  Sqrt/1 -> Relational Operator/1, Divide/2
  Constant1/1 -> Relational Operator/2
  Relational Operator/1 -> Switch/2
  Switch/1 -> Demux/1
  Demux/1 -> Ud/1
  Demux/2 -> Uq/1
  Mux/1 -> Divide/1, Gain3/1
  Gain3/1 -> Switch/1
  Divide/1 -> Switch/3
  [IdDem] -> Add/1
  [IdDem] -> Product1/1
  [IqDem] -> Product/2
  Add5/1 -> Sqrt/1

== system threelevel_12phase1/CurrentLoop/Subsystem/Subsystem/First_Order2 ==
  In1 : Inport
  Add : Sum
  Gain : Gain  Gain=2*pi*1e-6*100
  Gain1 : Gain  Gain=1-2*pi*1e-6*100
  Unit Delay : UnitDelay  SampleTime=-1  HasFrameUpgradeWarning=on
  ADC_temp : Outport
  wires:
  Add/1 -> ADC_temp/1, Gain1/1
  Gain1/1 -> Unit Delay/1
  Unit Delay/1 -> Add/2
  Gain/1 -> Add/1
  In1/1 -> Gain/1

== system threelevel_12phase1/CurrentLoop/Subsystem/Subsystem/针对负载波动的P增量 ==
  Abs : Abs
  Add4 : Sum  Inputs=+-
  Add7 : Sum
  Constant6 : Constant
  Delay : Delay  DelayLength=5
  Product2 : Product
  Step1 : Step  Time=0.5  Before=1  After=0.1  SampleTime=0
  Out1 : Outport
  wires:
  Constant6/1 -> Add7/1
  Add7/1 -> Out1/1
  Delay/1 -> Add4/2
  Product2/1 -> Add7/2
  [IqDem] -> Add4/1
  Step1/1 -> Product2/1
  Add4/1 -> Abs/1
  [IqDem] -> Delay/1
  Abs/1 -> Product2/2

== system threelevel_12phase1/CurrentLoop/Subsystem1/Subsystem/First_Order2 ==
  In1 : Inport
  Add : Sum
  Gain : Gain  Gain=2*pi*1e-6*100
  Gain1 : Gain  Gain=1-2*pi*1e-6*100
  Unit Delay : UnitDelay  SampleTime=-1  HasFrameUpgradeWarning=on
  ADC_temp : Outport
  wires:
  Add/1 -> ADC_temp/1, Gain1/1
  Gain1/1 -> Unit Delay/1
  Unit Delay/1 -> Add/2
  Gain/1 -> Add/1
  In1/1 -> Gain/1

== system threelevel_12phase1/CurrentLoop/Subsystem1/Subsystem/针对负载波动的P增量 ==
  Abs : Abs
  Add4 : Sum  Inputs=+-
  Add7 : Sum
  Constant6 : Constant
  Delay : Delay  DelayLength=5
  Product2 : Product
  Step1 : Step  Time=0.5  Before=1  After=0.1  SampleTime=0
  Out1 : Outport
  wires:
  Constant6/1 -> Add7/1
  Add7/1 -> Out1/1
  Delay/1 -> Add4/2
  Product2/1 -> Add7/2
  [IqDem] -> Add4/1
  Step1/1 -> Product2/1
  Add4/1 -> Abs/1
  [IqDem] -> Delay/1
  Abs/1 -> Product2/2

== system threelevel_12phase1/CurrentLoop/Subsystem2/Subsystem/First_Order2 ==
  In1 : Inport
  Add : Sum
  Gain : Gain  Gain=2*pi*1e-6*100
  Gain1 : Gain  Gain=1-2*pi*1e-6*100
  Unit Delay : UnitDelay  SampleTime=-1  HasFrameUpgradeWarning=on
  ADC_temp : Outport
  wires:
  Add/1 -> ADC_temp/1, Gain1/1
  Gain1/1 -> Unit Delay/1
  Unit Delay/1 -> Add/2
  Gain/1 -> Add/1
  In1/1 -> Gain/1

== system threelevel_12phase1/CurrentLoop/Subsystem2/Subsystem/针对负载波动的P增量 ==
  Abs : Abs
  Add4 : Sum  Inputs=+-
  Add7 : Sum
  Constant6 : Constant
  Delay : Delay  DelayLength=5
  Product2 : Product
  Step1 : Step  Time=0.5  Before=1  After=0.1  SampleTime=0
  Out1 : Outport
  wires:
  Constant6/1 -> Add7/1
  Add7/1 -> Out1/1
  Delay/1 -> Add4/2
  Product2/1 -> Add7/2
  [IqDem] -> Add4/1
  Step1/1 -> Product2/1
  Add4/1 -> Abs/1
  [IqDem] -> Delay/1
  Abs/1 -> Product2/2

== system threelevel_12phase1/CurrentLoop/Subsystem3/Subsystem/First_Order2 ==
  In1 : Inport
  Add : Sum
  Gain : Gain  Gain=2*pi*1e-6*100
  Gain1 : Gain  Gain=1-2*pi*1e-6*100
  Unit Delay : UnitDelay  SampleTime=-1  HasFrameUpgradeWarning=on
  ADC_temp : Outport
  wires:
  Add/1 -> ADC_temp/1, Gain1/1
  Gain1/1 -> Unit Delay/1
  Unit Delay/1 -> Add/2
  Gain/1 -> Add/1
  In1/1 -> Gain/1

== system threelevel_12phase1/CurrentLoop/Subsystem3/Subsystem/针对负载波动的P增量 ==
  Abs : Abs
  Add4 : Sum  Inputs=+-
  Add7 : Sum
  Constant6 : Constant
  Delay : Delay  DelayLength=5
  Product2 : Product
  Step1 : Step  Time=0.5  Before=1  After=0.1  SampleTime=0
  Out1 : Outport
  wires:
  Constant6/1 -> Add7/1
  Add7/1 -> Out1/1
  Delay/1 -> Add4/2
  Product2/1 -> Add7/2
  [IqDem] -> Add4/1
  Step1/1 -> Product2/1
  Add4/1 -> Abs/1
  [IqDem] -> Delay/1
  Abs/1 -> Product2/2
